simulink library "Lib_Solve_VectorCondition_TMATS"  (R2012b)
settings: Solver=ode45  StartTime=0.0  StopTime=10.0  RelTol=1e-3
undefined symbols (not defined in the file): MWS
Description:
  | Thomas Modules
settings Model: Creator=jwchapm2  LastModifiedBy=jwchapm2

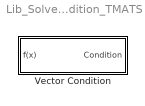
== system Lib_Solve_VectorCondition_TMATS ==
  Vector Condition : Subsystem  mask(T-MATS: Vector Condition Library Block){Cond_Limits_M=MWS.VCond.CondLim}
      mask prompts: Cond_Limits_M "Cond_Limits_M - Iteration Conditions Limits (nx1 or 1x1)"
      mask help:
      | Determines if the absolute value of each element in a vector is greater then a condition.
      | abs(V) > Cond_Limits
      | where V (nx1)and Cond_Limits (nx1 or 1x1)
      mask Help: web(which('Solver_TMATS_VC.html'),'-helpbrowser')

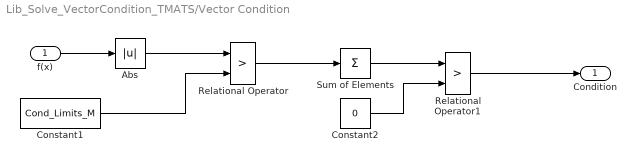
== system Lib_Solve_VectorCondition_TMATS/Vector Condition ==
  f(x) : Inport
  Abs : Abs
  Constant1 : Constant  Value=Cond_Limits_M
  Constant2 : Constant  Value=0
  Relational Operator : RelationalOperator  Operator=>  OutDataTypeStr=boolean
  Relational Operator1 : RelationalOperator  Operator=>  OutDataTypeStr=boolean
  Sum of Elements : Sum  Inputs=+
  Condition : Outport
  wires:
  Relational Operator1/1 -> Condition/1
  Sum of Elements/1 -> Relational Operator1/1
  Constant2/1 -> Relational Operator1/2
  Relational Operator/1 -> Sum of Elements/1
  f(x)/1 -> Abs/1
  Constant1/1 -> Relational Operator/2
  Abs/1 -> Relational Operator/1
